simulink model "Template_v3_08_2020a"  (R2020a)
settings: Solver=FixedStepAuto  StartTime=0.0  StopTime=tsim  FixedStep=baseRate  MaxStep=0.0001  RelTol=1e-6  AbsTol=1e-6  EnableMultiTasking=on
values from neighbouring files (symbols this model uses):
  baseRate = 0.05    [Run_Initializer.m]
  drop_states_ARM = [ pi/2, pi/2, 0]    [Run_Initializer.m]
  drop_states_BLACK = [ xLength/2, yLength/2, 0]    [Run_Initializer.m]
  drop_states_BLUE = [ xLength/2-0.5; yLength/2; 0]    [Run_Initializer.m]
  drop_states_RED = [ xLength/2+0.5, yLength/2, pi]    [Run_Initializer.m]
  F_Black_X_nominal = 0.2196    [Run_Initializer.m]
  F_Black_Y_nominal = 0.2825    [Run_Initializer.m]
  F_Blue_X_nominal = 0.2196    [Run_Initializer.m]
  F_Blue_Y_nominal = 0.2825    [Run_Initializer.m]
  F_red_X_nominal = 0.2196    [Run_Initializer.m]
  F_red_Y_nominal = 0.2825    [Run_Initializer.m]
  F_thrusters_BLACK = [F_Black_X_nominal; F_Black_X_nominal;                             F_Black_Y_nominal; F_Black_Y_nominal; F_Black_X_nominal;                              F_Black_X_nominal; F_Black_Y_nominal; F_Black_Y_nominal]    [Run_Initializer.m]
  F_thrusters_BLUE = [F_Blue_X_nominal; F_Blue_X_nominal;                             F_Blue_Y_nominal; F_Blue_Y_nominal; F_Blue_X_nominal;                              F_Blue_X_nominal; F_Blue_Y_nominal; F_Blue_Y_nominal]    [Run_Initializer.m]
  F_thrusters_RED = [F_red_X_nominal; F_red_X_nominal;                             F_red_Y_nominal; F_red_Y_nominal; F_red_X_nominal;                              F_red_X_nominal; F_red_Y_nominal; F_red_Y_nominal]    [Run_Initializer.m]
  Gamma1_el = 0.12    [Run_Initializer.m]
  Gamma1_sh = 0.005    [Run_Initializer.m]
  Gamma1_wr = 0.025    [Run_Initializer.m]
  Gamma2_el = 5    [Run_Initializer.m]
  Gamma2_sh = 15    [Run_Initializer.m]
  Gamma2_wr = 5    [Run_Initializer.m]
  Gamma3_el = 10    [Run_Initializer.m]
  Gamma3_sh = 40    [Run_Initializer.m]
  Gamma3_wr = 40    [Run_Initializer.m]
  Gamma4_el = 0.039    [Run_Initializer.m]
  Gamma4_sh = 0.015    [Run_Initializer.m]
  Gamma4_wr = 0.029    [Run_Initializer.m]
  Gamma5_el = 800    [Run_Initializer.m]
  Gamma5_sh = 800    [Run_Initializer.m]
  Gamma5_wr = 800    [Run_Initializer.m]
  Gamma6_el = 0.000001    (= 1e-06)    [Run_Initializer.m]
  Gamma6_sh = 0.005    [Run_Initializer.m]
  Gamma6_wr = 0.02    [Run_Initializer.m]
  home_states_BLACK = [ xLength/2; yLength/2; 0]    [Run_Initializer.m]
  home_states_BLUE = [ xLength/2-0.9; yLength/2; 0]    [Run_Initializer.m]
  home_states_RED = [ xLength/2+0.9; yLength/2; pi]    [Run_Initializer.m]
  init_states_BLACK = [ xLength/2; yLength/2; 0]    [Run_Initializer.m]
  init_states_BLUE = [ xLength/2-0.9; yLength/2; 0]    [Run_Initializer.m]
  init_states_RED = [ xLength/2+0.9; yLength/2; pi]    [Run_Initializer.m]
  Kd_tb = 1.0    (= 1)    [Run_Initializer.m]
  Kd_tblue = 1    [Run_Initializer.m]
  Kd_tr = 1.0    (= 1)    [Run_Initializer.m]
  Kd_xb = 8    [Run_Initializer.m]
  Kd_xblue = 8    [Run_Initializer.m]
  Kd_xr = 8    [Run_Initializer.m]
  Kd_yb = 8    [Run_Initializer.m]
  Kd_yblue = 8    [Run_Initializer.m]
  Kd_yr = 8    [Run_Initializer.m]
  Kp_tb = 0.1    [Run_Initializer.m]
  Kp_tblue = 0.1    [Run_Initializer.m]
  Kp_tr = 0.1    [Run_Initializer.m]
  Kp_xb = 2    [Run_Initializer.m]
  Kp_xblue = 2    [Run_Initializer.m]
  Kp_xr = 2    [Run_Initializer.m]
  Kp_yb = 2    [Run_Initializer.m]
  Kp_yblue = 2    [Run_Initializer.m]
  Kp_yr = 2    [Run_Initializer.m]
  noise_variance_BLACK = 0    [Run_Initializer.m]
  noise_variance_BLUE = 0    [Run_Initializer.m]
  noise_variance_RED = 0    [Run_Initializer.m]
  Phase0_End = Phase0_Duration    (= 10)    [Run_Initializer.m]
  Phase1_End = Phase0_Duration + Phase1_Duration    (= 15)    [Run_Initializer.m]
  Phase2_End = Phase0_Duration + Phase1_Duration +                                   Phase2_Duration    (= 35)    [Run_Initializer.m]
  Phase3_End = Phase0_Duration + Phase1_Duration +                                   Phase2_Duration + Phase3_Duration    (= 155)    [Run_Initializer.m]
  Phase3_SubPhase1_End = Phase2_End + Phase3_SubPhase1_Duration    (= 155)    [Run_Initializer.m]
  Phase3_SubPhase2_End = Phase2_End + Phase3_SubPhase1_Duration +                                   Phase3_SubPhase2_Duration    (= 155)    [Run_Initializer.m]
  Phase3_SubPhase3_End = Phase2_End + Phase3_SubPhase1_Duration +                                   Phase3_SubPhase2_Duration +                                  Phase3_SubPhase3_Duration    (= 155)    [Run_Initializer.m]
  Phase3_SubPhase4_End = Phase2_End + Phase3_SubPhase1_Duration +                                   Phase3_SubPhase2_Duration +                                  Phase3_SubPhase3_Duration +                                  Phase3_SubPhase4_Duration    [Run_Initializer.m]
  Phase4_End = Phase0_Duration + Phase1_Duration +                                   Phase2_Duration + Phase3_Duration +                                   Phase4_Duration    (= 275)    [Run_Initializer.m]
  Phase5_End = Phase0_Duration + Phase1_Duration +                                   Phase2_Duration + Phase3_Duration +                                   Phase4_Duration + Phase5_Duration    (= 295)    [Run_Initializer.m]
  thruster_dist2CG_BLACK = [72.80;-65.20;61.75;-79.75;65.20;-65.20;74.25;-54.75]    [Run_Initializer.m]
  thruster_dist2CG_BLUE = [83.10;-54.90;71.50;-70.00;54.90;-75.50;64.50;-64.50]    [Run_Initializer.m]
  thruster_dist2CG_RED = [69.38;-56.62;50.01;-81.49;61.12;-68.38;78.99;-52.01]    [Run_Initializer.m]
  Tz_lim_elarm = .1    (= 0.1)    [Run_Initializer.m]
  Tz_lim_sharm = .1    (= 0.1)    [Run_Initializer.m]
  Tz_lim_wrarm = .1    (= 0.1)    [Run_Initializer.m]
  xLength = 3.51155    [Run_Initializer.m]
  yLength = 2.41935    [Run_Initializer.m]
undefined symbols (not defined in the file or in its folder): b0, b1, b_out, CHASER_ABSOLUTE_POSITION, DiscIntNeverNeededParam, MAX_BODY_ANGULAR_VELOCITY, MAX_VELOCITY, model_param, platformSelection, relevant_half_range, relevant_state_mean, serverRate, simMode, w0, w1, w_out
libraries: dspstat3 x18, raspberrypiBasiclib x9, dspsigops x9, embdlinuxlib x7, simulink x7, MainLibrary x4, mspfiltlib x3, dsparch4 x3, etargetslib x1, sensehatlib x1
(part 5 of 12)

== system Template_v3_08_2020a/Phase #2: Move to Initial Position/Change RED Behavior/RED+ARM ==
  note: ARM Control Law - RED
  note: This section is reserved for any control law for the robotic manipulator.
  Action Port : ActionPort  ActionPortLabel=if(u1 == 4 | u1 == 5 | u1 == 10 | u1 == 11)
  Constant4 : Constant  Value=pi/2
  Constant5 : Constant  Value=pi/2
  Constant6 : Constant  Value=0
  Constant7 : Constant
  Data Store Write : DataStoreWrite  DataStoreName=RED_Shoulder_Command
  Data Store Write1 : DataStoreWrite  DataStoreName=RED_Elbow_Command
  Data Store Write2 : DataStoreWrite  DataStoreName=RED_Wrist_Command
  Data Store Write3 : DataStoreWrite  DataStoreName=RED_ARM_Control_Mode
  wires:
  Constant7/1 -> Data Store Write3/1
  Constant5/1 -> Data Store Write1/1
  Constant4/1 -> Data Store Write/1
  Constant6/1 -> Data Store Write2/1

== system Template_v3_08_2020a/Phase #3: Experiment/Change BLACK Behavior/Sub-Phase #1 ==
  note: PD Control Law - BLACK
  note: Additional Blocks
  note: A simple PD control law is used here to command the platform to it's initial position, as defined in the initializer.
  note: Additional blocks are stored here.
  Action Port : ActionPort  ActionPortLabel=if(u1 < u2)
  BLACK_Fx : DataStoreWrite  DataStoreName=BLACK_Fx
  BLACK_Fy : DataStoreWrite  DataStoreName=BLACK_Fy
  BLACK_Px : DataStoreRead  DataStoreName=BLACK_Px
  "BLACK_Py " : DataStoreRead  DataStoreName=BLACK_Py
  BLACK_Rz : DataStoreRead  DataStoreName=BLACK_Rz
  BLACK_RzD1 : Subsystem
  BLACK_Tz : DataStoreWrite  DataStoreName=BLACK_Tz
  Custom Discrete PD (Attitude) : Subsystem
  Custom Discrete PD (X-Position) : Subsystem
  Custom Discrete PD (Y-Position) : Subsystem
  Data Store Write3 : DataStoreWrite  DataStoreName=Float_State
  Desired X-Position (BLACK) : Constant  Value=xLength/2  SampleTime=-1
  Desired Y-Position (BLACK) : Constant  Value=yLength/2  SampleTime=-1
  Hough Control : Subsystem
  Puck State : Constant
  Subtract : Sum  Inputs=+-
  Subtract1 : Sum  Inputs=+-
  wires:
  Puck State/1 -> Data Store Write3/1
  "BLACK_Py "/1 -> Subtract1/2
  Desired X-Position (BLACK)/1 -> Subtract/1
  BLACK_RzD1/1(Out1) -> Hough Control/1(Ref)
  Custom Discrete PD (X-Position)/1(Fx) -> BLACK_Fx/1
  Desired Y-Position (BLACK)/1 -> Subtract1/1
  Hough Control/1(Err) -> Custom Discrete PD (Attitude)/1(ez)
  Subtract/1 -> Custom Discrete PD (X-Position)/1(ex)
  Custom Discrete PD (Y-Position)/1(Fy) -> BLACK_Fy/1
  Subtract1/1 -> Custom Discrete PD (Y-Position)/1(ey)
  Custom Discrete PD (Attitude)/1(Tz) -> BLACK_Tz/1
  BLACK_Rz/1 -> Hough Control/2(Act)
  BLACK_Px/1 -> Subtract/2

== system Template_v3_08_2020a/Phase #3: Experiment/Change BLACK Behavior/Sub-Phase #2  ==
  note: PD Control Law - BLACK
  note: Additional Blocks
  note: Additional blocks are stored here.
  Action Port : ActionPort  ActionPortLabel=elseif(u1 < u3)
  BLACK_Fx : DataStoreWrite  DataStoreName=BLACK_Fx
  BLACK_Fy : DataStoreWrite  DataStoreName=BLACK_Fy
  BLACK_Px : DataStoreRead  DataStoreName=BLACK_Px
  "BLACK_Py " : DataStoreRead  DataStoreName=BLACK_Py
  BLACK_Rz : DataStoreRead  DataStoreName=BLACK_Rz
  BLACK_RzD1 : Subsystem
  BLACK_Tz : DataStoreWrite  DataStoreName=BLACK_Tz
  Custom Discrete PD (Attitude) : Subsystem
  Custom Discrete PD (X-Position) : Subsystem
  Custom Discrete PD (Y-Position) : Subsystem
  Data Store Write3 : DataStoreWrite  DataStoreName=Float_State
  Desired X-Position (BLACK) : Constant  Value=xLength/2  SampleTime=-1
  Desired Y-Position (BLACK) : Constant  Value=yLength/2  SampleTime=-1
  Hough Control : Subsystem
  Puck State : Constant
  Subtract : Sum  Inputs=+-
  Subtract1 : Sum  Inputs=+-
  wires:
  Puck State/1 -> Data Store Write3/1
  BLACK_Px/1 -> Subtract/2
  Custom Discrete PD (Y-Position)/1(Fy) -> BLACK_Fy/1
  Subtract/1 -> Custom Discrete PD (X-Position)/1(ex)
  Desired Y-Position (BLACK)/1 -> Subtract1/1
  Custom Discrete PD (Attitude)/1(Tz) -> BLACK_Tz/1
  Subtract1/1 -> Custom Discrete PD (Y-Position)/1(ey)
  BLACK_Rz/1 -> Hough Control/2(Act)
  Custom Discrete PD (X-Position)/1(Fx) -> BLACK_Fx/1
  Hough Control/1(Err) -> Custom Discrete PD (Attitude)/1(ez)
  "BLACK_Py "/1 -> Subtract1/2
  Desired X-Position (BLACK)/1 -> Subtract/1
  BLACK_RzD1/1(Out1) -> Hough Control/1(Ref)

== system Template_v3_08_2020a/Phase #3: Experiment/Change BLACK Behavior/Sub-Phase #3  ==
  note: PD Control Law - BLACK
  note: Additional Blocks
  note: Additional blocks are stored here.
  Action Port : ActionPort  ActionPortLabel=elseif( u1 < u4)
  BLACK_Fx : DataStoreWrite  DataStoreName=BLACK_Fx
  BLACK_Fy : DataStoreWrite  DataStoreName=BLACK_Fy
  BLACK_Px : DataStoreRead  DataStoreName=BLACK_Px
  "BLACK_Py " : DataStoreRead  DataStoreName=BLACK_Py
  BLACK_Rz : DataStoreRead  DataStoreName=BLACK_Rz
  BLACK_RzD1 : Subsystem
  BLACK_Tz : DataStoreWrite  DataStoreName=BLACK_Tz
  Custom Discrete PD (Attitude) : Subsystem
  Custom Discrete PD (X-Position) : Subsystem
  Custom Discrete PD (Y-Position) : Subsystem
  Data Store Write3 : DataStoreWrite  DataStoreName=Float_State
  Desired X-Position (BLACK) : Constant  Value=xLength/2  SampleTime=-1
  Desired Y-Position (BLACK) : Constant  Value=yLength/2  SampleTime=-1
  Hough Control : Subsystem
  Puck State : Constant
  Subtract : Sum  Inputs=+-
  Subtract1 : Sum  Inputs=+-
  wires:
  Puck State/1 -> Data Store Write3/1
  BLACK_Px/1 -> Subtract/2
  Custom Discrete PD (Y-Position)/1(Fy) -> BLACK_Fy/1
  Subtract/1 -> Custom Discrete PD (X-Position)/1(ex)
  Desired Y-Position (BLACK)/1 -> Subtract1/1
  Custom Discrete PD (Attitude)/1(Tz) -> BLACK_Tz/1
  Subtract1/1 -> Custom Discrete PD (Y-Position)/1(ey)
  BLACK_Rz/1 -> Hough Control/2(Act)
  Custom Discrete PD (X-Position)/1(Fx) -> BLACK_Fx/1
  Hough Control/1(Err) -> Custom Discrete PD (Attitude)/1(ez)
  "BLACK_Py "/1 -> Subtract1/2
  Desired X-Position (BLACK)/1 -> Subtract/1
  BLACK_RzD1/1(Out1) -> Hough Control/1(Ref)

== system Template_v3_08_2020a/Phase #3: Experiment/Change BLACK Behavior/Sub-Phase #4 ==
  note: PD Control Law - BLACK
  note: Additional Blocks
  note: A simple PD control law is used here to command the platform to it's initial position, as defined in the initializer.
  note: Additional blocks are stored here.
  Action Port : ActionPort  ActionPortLabel=elseif( u1 < u5)
  BLACK_Fx : DataStoreWrite  DataStoreName=BLACK_Fx
  BLACK_Fy : DataStoreWrite  DataStoreName=BLACK_Fy
  BLACK_Px : DataStoreRead  DataStoreName=BLACK_Px
  "BLACK_Py " : DataStoreRead  DataStoreName=BLACK_Py
  BLACK_Rz : DataStoreRead  DataStoreName=BLACK_Rz
  BLACK_RzD : Subsystem  Commented=on
  BLACK_RzD1 : Subsystem
  BLACK_Tz : DataStoreWrite  DataStoreName=BLACK_Tz
  Custom Discrete PD (Attitude) : Subsystem
  Custom Discrete PD (X-Position) : Subsystem
  Custom Discrete PD (Y-Position) : Subsystem
  Data Store Write3 : DataStoreWrite  DataStoreName=Float_State
  Desired X-Position (BLACK) : Constant  Value=xLength/2  SampleTime=-1
  Desired Y-Position (BLACK) : Constant  Value=yLength/2  SampleTime=-1
  Hough Control : Subsystem
  Puck State : Constant
  Subtract : Sum  Inputs=+-
  Subtract1 : Sum  Inputs=+-
  wires:
  Puck State/1 -> Data Store Write3/1
  BLACK_Px/1 -> Subtract/2
  Custom Discrete PD (Y-Position)/1(Fy) -> BLACK_Fy/1
  Subtract/1 -> Custom Discrete PD (X-Position)/1(ex)
  Desired Y-Position (BLACK)/1 -> Subtract1/1
  Custom Discrete PD (Attitude)/1(Tz) -> BLACK_Tz/1
  Subtract1/1 -> Custom Discrete PD (Y-Position)/1(ey)
  BLACK_Rz/1 -> Hough Control/2(Act)
  Custom Discrete PD (X-Position)/1(Fx) -> BLACK_Fx/1
  Hough Control/1(Err) -> Custom Discrete PD (Attitude)/1(ez)
  "BLACK_Py "/1 -> Subtract1/2
  Desired X-Position (BLACK)/1 -> Subtract/1
  BLACK_RzD1/1(Out1) -> Hough Control/1(Ref)

== system Template_v3_08_2020a/Phase #3: Experiment/Change BLACK Behavior/Subsystem ==
  Universal_Time : DataStoreRead  DataStoreName=Univ_Time
  Time : Outport  VectorParamsAs1DForOutWhenUnconnected=off
  wires:
  Universal_Time/1 -> Time/1

== system Template_v3_08_2020a/Phase #3: Experiment/Change BLUE Behavior/Sub-Phase #1 ==
  note: PD Control Law - BLUE
  note: A simple PD control law is used here to command the platform to it's initial position, as defined in the initializer.
  note: Additional Blocks
  note: Additional blocks are stored here.
  Action Port : ActionPort  ActionPortLabel=if(u1 < u2)
  BLUE_Fx : DataStoreWrite  DataStoreName=BLUE_Fx
  BLUE_Fy : DataStoreWrite  DataStoreName=BLUE_Fy
  BLUE_Px : DataStoreRead  DataStoreName=BLUE_Px
  "BLUE_Py " : DataStoreRead  DataStoreName=BLUE_Py
  BLUE_Rz : DataStoreRead  DataStoreName=BLUE_Rz
  BLUE_Tz : DataStoreWrite  DataStoreName=BLUE_Tz
  Custom Discrete PD (Attitude) : Subsystem
  Custom Discrete PD (X-Position) : Subsystem
  Custom Discrete PD (Y-Position) : Subsystem
  Data Store Write1 : DataStoreWrite  DataStoreName=Float_State
  Hough Control : Subsystem
  MATLAB Function2 : MATLAB Function  TreatAsAtomicUnit=on
  MATLAB Function3 : MATLAB Function  TreatAsAtomicUnit=on
  Puck State : Constant
  RED_Rz_REF1 : Subsystem
  Subsystem2 : Subsystem
  Subtract : Sum  Inputs=+-
  Subtract1 : Sum  Inputs=+-
  wires:
  Puck State/1 -> Data Store Write1/1
  Subtract/1 -> Custom Discrete PD (X-Position)/1(ex)
  Custom Discrete PD (X-Position)/1(Fx) -> BLUE_Fx/1
  Subtract1/1 -> Custom Discrete PD (Y-Position)/1(ey)
  Hough Control/1(Err) -> Custom Discrete PD (Attitude)/1(ez)
  Custom Discrete PD (Attitude)/1(Tz) -> BLUE_Tz/1
  Custom Discrete PD (Y-Position)/1(Fy) -> BLUE_Fy/1
  MATLAB Function3/1(y) -> Subtract1/1
  BLUE_Px/1 -> Subtract/2
  MATLAB Function2/1(x) -> Subtract/1
  Subsystem2/1(Out1) -> MATLAB Function2/1(t), MATLAB Function3/1(t)
  "BLUE_Py "/1 -> Subtract1/2
  RED_Rz_REF1/1(Ref) -> Hough Control/1(Ref)
  BLUE_Rz/1 -> Hough Control/2(Act)

== system Template_v3_08_2020a/Phase #3: Experiment/Change BLUE Behavior/Sub-Phase #2  ==
  note: Additional blocks are stored here.
  note: A simple PD control law is used here to command the platform to it's initial position, as defined in the initializer.
  note: Additional Blocks
  note: PD Control Law - BLUE
  Action Port : ActionPort  ActionPortLabel=elseif(u1 < u3)
  BLUE_Fx : DataStoreWrite  DataStoreName=BLUE_Fx
  BLUE_Fy : DataStoreWrite  DataStoreName=BLUE_Fy
  BLUE_Px : DataStoreRead  DataStoreName=BLUE_Px
  "BLUE_Py " : DataStoreRead  DataStoreName=BLUE_Py
  BLUE_Rz : DataStoreRead  DataStoreName=BLUE_Rz
  BLUE_Tz : DataStoreWrite  DataStoreName=BLUE_Tz
  Custom Discrete PD (Attitude) : Subsystem
  Custom Discrete PD (X-Position) : Subsystem
  Custom Discrete PD (Y-Position) : Subsystem
  Data Store Write1 : DataStoreWrite  DataStoreName=Float_State
  Hough Control : Subsystem
  MATLAB Function2 : MATLAB Function  TreatAsAtomicUnit=on
  MATLAB Function3 : MATLAB Function  TreatAsAtomicUnit=on
  Puck State : Constant
  RED_Rz_REF1 : Subsystem
  Subsystem2 : Subsystem
  Subtract : Sum  Inputs=+-
  Subtract1 : Sum  Inputs=+-
  wires:
  Puck State/1 -> Data Store Write1/1
  BLUE_Rz/1 -> Hough Control/2(Act)
  RED_Rz_REF1/1(Ref) -> Hough Control/1(Ref)
  Custom Discrete PD (Y-Position)/1(Fy) -> BLUE_Fy/1
  Subtract/1 -> Custom Discrete PD (X-Position)/1(ex)
  Subtract1/1 -> Custom Discrete PD (Y-Position)/1(ey)
  BLUE_Px/1 -> Subtract/2
  Custom Discrete PD (X-Position)/1(Fx) -> BLUE_Fx/1
  "BLUE_Py "/1 -> Subtract1/2
  Subsystem2/1(Out1) -> MATLAB Function2/1(t), MATLAB Function3/1(t)
  MATLAB Function2/1(x) -> Subtract/1
  Hough Control/1(Err) -> Custom Discrete PD (Attitude)/1(ez)
  MATLAB Function3/1(y) -> Subtract1/1
  Custom Discrete PD (Attitude)/1(Tz) -> BLUE_Tz/1

== system Template_v3_08_2020a/Phase #3: Experiment/Change BLUE Behavior/Sub-Phase #3  ==
  note: Additional blocks are stored here.
  note: A simple PD control law is used here to command the platform to it's initial position, as defined in the initializer.
  note: Additional Blocks
  note: PD Control Law - BLUE
  Action Port : ActionPort  ActionPortLabel=elseif( u1 < u4)
  BLUE_Fx : DataStoreWrite  DataStoreName=BLUE_Fx
  BLUE_Fy : DataStoreWrite  DataStoreName=BLUE_Fy
  BLUE_Px : DataStoreRead  DataStoreName=BLUE_Px
  "BLUE_Py " : DataStoreRead  DataStoreName=BLUE_Py
  BLUE_Rz : DataStoreRead  DataStoreName=BLUE_Rz
  BLUE_Tz : DataStoreWrite  DataStoreName=BLUE_Tz
  Custom Discrete PD (Attitude) : Subsystem
  Custom Discrete PD (X-Position) : Subsystem
  Custom Discrete PD (Y-Position) : Subsystem
  Data Store Write1 : DataStoreWrite  DataStoreName=Float_State
  Hough Control : Subsystem
  MATLAB Function2 : MATLAB Function  TreatAsAtomicUnit=on
  MATLAB Function3 : MATLAB Function  TreatAsAtomicUnit=on
  Puck State : Constant
  RED_Rz_REF1 : Subsystem
  Subsystem2 : Subsystem
  Subtract : Sum  Inputs=+-
  Subtract1 : Sum  Inputs=+-
  wires:
  Puck State/1 -> Data Store Write1/1
  BLUE_Rz/1 -> Hough Control/2(Act)
  RED_Rz_REF1/1(Ref) -> Hough Control/1(Ref)
  Custom Discrete PD (Y-Position)/1(Fy) -> BLUE_Fy/1
  Subtract/1 -> Custom Discrete PD (X-Position)/1(ex)
  Subtract1/1 -> Custom Discrete PD (Y-Position)/1(ey)
  BLUE_Px/1 -> Subtract/2
  Custom Discrete PD (X-Position)/1(Fx) -> BLUE_Fx/1
  "BLUE_Py "/1 -> Subtract1/2
  Subsystem2/1(Out1) -> MATLAB Function2/1(t), MATLAB Function3/1(t)
  MATLAB Function2/1(x) -> Subtract/1
  Hough Control/1(Err) -> Custom Discrete PD (Attitude)/1(ez)
  MATLAB Function3/1(y) -> Subtract1/1
  Custom Discrete PD (Attitude)/1(Tz) -> BLUE_Tz/1

== system Template_v3_08_2020a/Phase #3: Experiment/Change BLUE Behavior/Sub-Phase #4 ==
  note: Additional blocks are stored here.
  note: A simple PD control law is used here to command the platform to it's initial position, as defined in the initializer.
  note: Additional Blocks
  note: PD Control Law - BLUE
  Action Port : ActionPort  ActionPortLabel=elseif( u1 < u5)
  BLUE_Fx : DataStoreWrite  DataStoreName=BLUE_Fx
  BLUE_Fy : DataStoreWrite  DataStoreName=BLUE_Fy
  BLUE_Px : DataStoreRead  DataStoreName=BLUE_Px
  "BLUE_Py " : DataStoreRead  DataStoreName=BLUE_Py
  BLUE_Rz : DataStoreRead  DataStoreName=BLUE_Rz
  BLUE_Tz : DataStoreWrite  DataStoreName=BLUE_Tz
  Custom Discrete PD (Attitude) : Subsystem
  Custom Discrete PD (X-Position) : Subsystem
  Custom Discrete PD (Y-Position) : Subsystem
  Data Store Write1 : DataStoreWrite  DataStoreName=Float_State
  Hough Control : Subsystem
  MATLAB Function2 : MATLAB Function  TreatAsAtomicUnit=on
  MATLAB Function3 : MATLAB Function  TreatAsAtomicUnit=on
  Puck State : Constant
  RED_Rz_REF1 : Subsystem
  Subsystem2 : Subsystem
  Subtract : Sum  Inputs=+-
  Subtract1 : Sum  Inputs=+-
  wires:
  Puck State/1 -> Data Store Write1/1
  BLUE_Rz/1 -> Hough Control/2(Act)
  RED_Rz_REF1/1(Ref) -> Hough Control/1(Ref)
  Custom Discrete PD (Y-Position)/1(Fy) -> BLUE_Fy/1
  Subtract/1 -> Custom Discrete PD (X-Position)/1(ex)
  Subtract1/1 -> Custom Discrete PD (Y-Position)/1(ey)
  BLUE_Px/1 -> Subtract/2
  Custom Discrete PD (X-Position)/1(Fx) -> BLUE_Fx/1
  "BLUE_Py "/1 -> Subtract1/2
  Subsystem2/1(Out1) -> MATLAB Function2/1(t), MATLAB Function3/1(t)
  MATLAB Function2/1(x) -> Subtract/1
  Hough Control/1(Err) -> Custom Discrete PD (Attitude)/1(ez)
  MATLAB Function3/1(y) -> Subtract1/1
  Custom Discrete PD (Attitude)/1(Tz) -> BLUE_Tz/1

== system Template_v3_08_2020a/Phase #3: Experiment/Change BLUE Behavior/Subsystem ==
  Universal_Time : DataStoreRead  DataStoreName=Univ_Time
  Time : Outport  VectorParamsAs1DForOutWhenUnconnected=off
  wires:
  Universal_Time/1 -> Time/1

== system Template_v3_08_2020a/Phase #3: Experiment/Change RED Behavior/Sub-Phase #1 ==
  note: PD Control Law - RED
  note: Additional Blocks
  note: Additional blocks are stored above. Note that to control attitude using the RW, simply replace RED_Tz with RED_Tz_RW.
  note: A simple PD control law is used here to command the platform to it's initial position, as defined in the initializer.
  note: ARM Control Law - RED
  Action Port : ActionPort  ActionPortLabel=if(u1 < u2)
  Constant1 : Constant  Value=0
  Constant4 : Constant  Value=platformSelection
  Custom Discrete PD (Attitude) : Subsystem
  Custom Discrete PD (X-Position) : Subsystem
  Custom Discrete PD (Y-Position) : Subsystem
  Data Store Write3 : DataStoreWrite  DataStoreName=Float_State
  Hough Control : Subsystem
  If : If  IfExpression=u1 == 4 | u1 == 5 | u1 == 10 | u1 == 11
  MATLAB Function : MATLAB Function  TreatAsAtomicUnit=on
  MATLAB Function1 : MATLAB Function  TreatAsAtomicUnit=on
  Puck State : Constant
  RED : Subsystem  TreatAsAtomicUnit=on
  RED+ARM : Subsystem  TreatAsAtomicUnit=on
  RED_Fx : DataStoreWrite  DataStoreName=RED_Fx
  RED_Fy : DataStoreWrite  DataStoreName=RED_Fy
  RED_Px3 : DataStoreRead  DataStoreName=RED_Px
  "RED_Py " : DataStoreRead  DataStoreName=RED_Py
  RED_Rz : DataStoreRead  DataStoreName=RED_Rz
  RED_RzD : Subsystem
  RED_Tz : DataStoreWrite  DataStoreName=RED_Tz
  RED_Tz_RW : DataStoreWrite  DataStoreName=RED_Tz_RW
  Subsystem1 : Subsystem
  Subtract : Sum  Inputs=+-
  Subtract1 : Sum  Inputs=+-
  wires:
  Constant1/1 -> RED_Tz_RW/1
  Puck State/1 -> Data Store Write3/1
  Custom Discrete PD (Y-Position)/1(Fy) -> RED_Fy/1
  Custom Discrete PD (X-Position)/1(Fx) -> RED_Fx/1
  Custom Discrete PD (Attitude)/1(Tz) -> RED_Tz/1
  Hough Control/1(Err) -> Custom Discrete PD (Attitude)/1(ez)
  Subsystem1/1(Out1) -> MATLAB Function/1(t), MATLAB Function1/1(t)
  RED_Px3/1 -> Subtract/2
  MATLAB Function1/1(y) -> Subtract1/1
  "RED_Py "/1 -> Subtract1/2
  MATLAB Function/1(x) -> Subtract/1
  Subtract/1 -> Custom Discrete PD (X-Position)/1(ex)
  RED_Rz/1 -> Hough Control/2(Act)
  Subtract1/1 -> Custom Discrete PD (Y-Position)/1(ey)
  RED_RzD/1(Ref) -> Hough Control/1(Ref)
  If/1 -> RED+ARM/Action
  Constant4/1 -> If/1
  If/2 -> RED/Action

== system Template_v3_08_2020a/Phase #3: Experiment/Change RED Behavior/Sub-Phase #2  ==
  note: PD Control Law - RED
  note: Additional Blocks
  note: Additional blocks are stored above. Note that to control attitude using the RW, simply replace RED_Tz with RED_Tz_RW.
  note: ARM Control Law - RED
  Action Port : ActionPort  ActionPortLabel=elseif(u1 < u3)
  BLACK_RzD1 : Subsystem
  Constant1 : Constant  Value=0
  Constant4 : Constant  Value=platformSelection
  Custom Discrete PD (Attitude) : Subsystem
  Custom Discrete PD (X-Position) : Subsystem
  Custom Discrete PD (Y-Position) : Subsystem
  Data Store Write3 : DataStoreWrite  DataStoreName=Float_State
  Hough Control : Subsystem
  If : If  IfExpression=u1 == 4 | u1 == 5 | u1 == 10 | u1 == 11
  MATLAB Function : MATLAB Function  TreatAsAtomicUnit=on
  MATLAB Function1 : MATLAB Function  TreatAsAtomicUnit=on
  Puck State : Constant
  RED : Subsystem  TreatAsAtomicUnit=on
  RED+ARM : Subsystem  TreatAsAtomicUnit=on
  RED_Fx : DataStoreWrite  DataStoreName=RED_Fx
  RED_Fy : DataStoreWrite  DataStoreName=RED_Fy
  RED_Px1 : DataStoreRead  DataStoreName=RED_Px
  "RED_Py " : DataStoreRead  DataStoreName=RED_Py
  RED_Rz : DataStoreRead  DataStoreName=RED_Rz
  RED_Tz : DataStoreWrite  DataStoreName=RED_Tz
  RED_Tz_RW : DataStoreWrite  DataStoreName=RED_Tz_RW
  Subsystem1 : Subsystem
  Subtract : Sum  Inputs=+-
  Subtract2 : Sum  Inputs=+-
  wires:
  Constant1/1 -> RED_Tz_RW/1
  Puck State/1 -> Data Store Write3/1
  Subtract2/1 -> Custom Discrete PD (Y-Position)/1(ey)
  "RED_Py "/1 -> Subtract2/2
  BLACK_RzD1/1(Ref) -> Hough Control/1(Ref)
  MATLAB Function/1(x) -> Subtract/1
  RED_Rz/1 -> Hough Control/2(Act)
  Subtract/1 -> Custom Discrete PD (X-Position)/1(ex)
  MATLAB Function1/1(y) -> Subtract2/1
  Custom Discrete PD (Attitude)/1(Tz) -> RED_Tz/1
  RED_Px1/1 -> Subtract/2
  Subsystem1/1(Out1) -> MATLAB Function/1(t), MATLAB Function1/1(t)
  Custom Discrete PD (X-Position)/1(Fx) -> RED_Fx/1
  Hough Control/1(Err) -> Custom Discrete PD (Attitude)/1(ez)
  Custom Discrete PD (Y-Position)/1(Fy) -> RED_Fy/1
  If/1 -> RED+ARM/Action
  Constant4/1 -> If/1
  If/2 -> RED/Action

== system Template_v3_08_2020a/Phase #3: Experiment/Change RED Behavior/Sub-Phase #3  ==
  note: PD Control Law - RED
  note: Additional Blocks
  note: Additional blocks are stored above. Note that to control attitude using the RW, simply replace RED_Tz with RED_Tz_RW.
  note: ARM Control Law - RED
  Action Port : ActionPort  ActionPortLabel=elseif( u1 < u4)
  Constant1 : Constant  Value=platformSelection
  Constant4 : Constant  Value=0
  Custom Discrete PD (Attitude) : Subsystem  Commented=on
  Custom Discrete PD (X-Position) : Subsystem
  Custom Discrete PD (Y-Position) : Subsystem
  Data Store Write3 : DataStoreWrite  DataStoreName=Float_State
  Hough Control : Subsystem  Commented=on
  If : If  IfExpression=u1 == 4 | u1 == 5 | u1 == 10 | u1 == 11
  MATLAB Function : MATLAB Function  TreatAsAtomicUnit=on
  MATLAB Function1 : MATLAB Function  TreatAsAtomicUnit=on
  Puck State : Constant
  RED : Subsystem  TreatAsAtomicUnit=on
  RED+ARM : Subsystem  TreatAsAtomicUnit=on
  RED_Fx : DataStoreWrite  DataStoreName=RED_Fx
  RED_Fy : DataStoreWrite  DataStoreName=RED_Fy
  RED_Px1 : DataStoreRead  DataStoreName=RED_Px
  "RED_Py " : DataStoreRead  DataStoreName=RED_Py
  RED_Rz : DataStoreRead  Commented=on  DataStoreName=RED_Rz
  RED_Rz_REF : Subsystem  Commented=on
  RED_Tz : DataStoreWrite  Commented=on  DataStoreName=RED_Tz
  RED_Tz_RW : DataStoreWrite  DataStoreName=RED_Tz_RW
  Saturation : Saturate  UpperLimit=Tz_lim_sharm  LowerLimit=-Tz_lim_sharm
  Saturation1 : Saturate  UpperLimit=Tz_lim_elarm  LowerLimit=-Tz_lim_elarm
  Saturation3 : Saturate  UpperLimit=Tz_lim_wrarm  LowerLimit=-Tz_lim_wrarm
  Subsystem1 : Subsystem
  Subtract : Sum  Inputs=+-
  Subtract2 : Sum  Inputs=+-
  wires:
  Puck State/1 -> Data Store Write3/1
  Hough Control/1(Err) -> Custom Discrete PD (Attitude)/1(ez)
  Custom Discrete PD (Y-Position)/1(Fy) -> RED_Fy/1
  Custom Discrete PD (X-Position)/1(Fx) -> RED_Fx/1
  RED_Rz/1 -> Hough Control/2(Act)
  MATLAB Function1/1(y) -> Subtract2/1
  Custom Discrete PD (Attitude)/1(Tz) -> RED_Tz/1
  MATLAB Function/1(x) -> Subtract/1
  Subtract/1 -> Custom Discrete PD (X-Position)/1(ex)
  "RED_Py "/1 -> Subtract2/2
  RED_Rz_REF/1(Ref) -> Hough Control/1(Ref)
  RED_Px1/1 -> Subtract/2
  Subsystem1/1(Out1) -> MATLAB Function/1(t), MATLAB Function1/1(t)
  Subtract2/1 -> Custom Discrete PD (Y-Position)/1(ey)
  Constant4/1 -> RED_Tz_RW/1
  If/1 -> RED+ARM/Action
  Constant1/1 -> If/1
  If/2 -> RED/Action

== system Template_v3_08_2020a/Phase #3: Experiment/Change RED Behavior/Sub-Phase #4 ==
  note: PD Control Law - RED
  note: Additional Blocks
  note: Additional blocks are stored above. Note that to control attitude using the RW, simply replace RED_Tz with RED_Tz_RW.
  note: A simple PD control law is used here to command the platform to it's initial position, as defined in the initializer.
  note: ARM Control Law - RED
  Action Port : ActionPort  ActionPortLabel=elseif( u1 < u5)
  Constant1 : Constant  Value=0
  Constant3 : Constant  Value=platformSelection
  Custom Discrete PD (Attitude) : Subsystem
  Custom Discrete PD (X-Position) : Subsystem
  Custom Discrete PD (Y-Position) : Subsystem
  Data Store Write3 : DataStoreWrite  DataStoreName=Float_State
  Hough Control : Subsystem
  If : If  IfExpression=u1 == 4 | u1 == 5 | u1 == 10 | u1 == 11
  MATLAB Function : MATLAB Function  TreatAsAtomicUnit=on
  MATLAB Function1 : MATLAB Function  TreatAsAtomicUnit=on
  Puck State : Constant
  RED : Subsystem  TreatAsAtomicUnit=on
  RED+ARM : Subsystem  TreatAsAtomicUnit=on
  RED_Fx : DataStoreWrite  DataStoreName=RED_Fx
  RED_Fy : DataStoreWrite  DataStoreName=RED_Fy
  RED_Px1 : DataStoreRead  DataStoreName=RED_Px
  "RED_Py " : DataStoreRead  DataStoreName=RED_Py
  RED_Rz : DataStoreRead  DataStoreName=RED_Rz
  RED_Rz_REF : Subsystem
  RED_Tz : DataStoreWrite  DataStoreName=RED_Tz
  RED_Tz_RW : DataStoreWrite  DataStoreName=RED_Tz_RW
  Subsystem1 : Subsystem
  Subtract : Sum  Inputs=+-
  Subtract1 : Sum  Inputs=+-
  wires:
  Constant1/1 -> RED_Tz_RW/1
  RED_Rz/1 -> Hough Control/2(Act)
  Subtract/1 -> Custom Discrete PD (X-Position)/1(ex)
  Custom Discrete PD (X-Position)/1(Fx) -> RED_Fx/1
  Custom Discrete PD (Y-Position)/1(Fy) -> RED_Fy/1
  RED_Px1/1 -> Subtract/2
  Custom Discrete PD (Attitude)/1(Tz) -> RED_Tz/1
  "RED_Py "/1 -> Subtract1/2
  Hough Control/1(Err) -> Custom Discrete PD (Attitude)/1(ez)
  Subtract1/1 -> Custom Discrete PD (Y-Position)/1(ey)
  Puck State/1 -> Data Store Write3/1
  Subsystem1/1(Out1) -> MATLAB Function/1(t), MATLAB Function1/1(t)
  MATLAB Function/1(x) -> Subtract/1
  MATLAB Function1/1(y) -> Subtract1/1
  RED_Rz_REF/1(Ref) -> Hough Control/1(Ref)
  If/2 -> RED/Action
  If/1 -> RED+ARM/Action
  Constant3/1 -> If/1

== system Template_v3_08_2020a/Phase #3: Experiment/Change RED Behavior/Subsystem ==
  Universal_Time : DataStoreRead  DataStoreName=Univ_Time
  Time : Outport  VectorParamsAs1DForOutWhenUnconnected=off
  wires:
  Universal_Time/1 -> Time/1

== system Template_v3_08_2020a/Phase #4: Return Home/Change BLACK Behavior/Custom Discrete PD (Attitude) ==
  ez : Inport
  Sum3 : Sum
  kd_tb : Gain  Gain=Kd_tb
  kp_tb : Gain  Gain=Kp_tb
  "x_dot -> x1" : Subsystem
  Tz : Outport  VectorParamsAs1DForOutWhenUnconnected=off
  wires:
  kd_tb/1 -> Sum3/1
  Sum3/1 -> Tz/1
  kp_tb/1 -> Sum3/2
  "x_dot -> x1"/1(dy(t)/dt) -> kd_tb/1
  ez/1 -> "x_dot -> x1"/1(y(t)), kp_tb/1

== system Template_v3_08_2020a/Phase #4: Return Home/Change BLACK Behavior/Custom Discrete PD (X-Position) ==
  ex : Inport
  Sum3 : Sum
  kd_xb : Gain  Gain=Kd_xb
  kp_xb : Gain  Gain=Kp_xb
  "x_dot -> x1" : Subsystem
  Fx : Outport  VectorParamsAs1DForOutWhenUnconnected=off
  wires:
  kd_xb/1 -> Sum3/1
  ex/1 -> "x_dot -> x1"/1(y(t)), kp_xb/1
  kp_xb/1 -> Sum3/2
  "x_dot -> x1"/1(dy(t)/dt) -> kd_xb/1
  Sum3/1 -> Fx/1

== system Template_v3_08_2020a/Phase #4: Return Home/Change BLACK Behavior/Custom Discrete PD (Y-Position) ==
  ey : Inport
  Sum3 : Sum
  kd_yb : Gain  Gain=Kd_yb
  kp_yb : Gain  Gain=Kp_yb
  "x_dot -> x1" : Subsystem
  Fy : Outport  VectorParamsAs1DForOutWhenUnconnected=off
  wires:
  kd_yb/1 -> Sum3/1
  Sum3/1 -> Fy/1
  kp_yb/1 -> Sum3/2
  "x_dot -> x1"/1(dy(t)/dt) -> kd_yb/1
  ey/1 -> "x_dot -> x1"/1(y(t)), kp_yb/1

== system Template_v3_08_2020a/Phase #4: Return Home/Change BLACK Behavior/Hough Control ==
  Ref : Inport
  Act : Inport  Port=2
  MATLAB Function2 : MATLAB Function  TreatAsAtomicUnit=on
  MATLAB Function3 : MATLAB Function  TreatAsAtomicUnit=on
  MATLAB Function4 : MATLAB Function  TreatAsAtomicUnit=on
  Subtract2 : Sum  Inputs=+-
  Err : Outport  VectorParamsAs1DForOutWhenUnconnected=off
  wires:
  MATLAB Function4/1(e_out) -> Err/1
  MATLAB Function2/1(Oy) -> MATLAB Function4/1(Oy)
  Subtract2/1 -> MATLAB Function4/2(e_in)
  MATLAB Function2/2(Ox) -> Subtract2/1
  Act/1 -> MATLAB Function3/1(z)
  Ref/1 -> MATLAB Function2/1(z)
  MATLAB Function3/1(Ox) -> Subtract2/2

== system Template_v3_08_2020a/Phase #4: Return Home/Change BLUE Behavior/Custom Discrete PD (Attitude) ==
  ez : Inport
  Sum3 : Sum
  kd_tb : Gain  Gain=Kd_tblue
  kp_tb : Gain  Gain=Kp_tblue
  "x_dot -> x1" : Subsystem
  Tz : Outport  VectorParamsAs1DForOutWhenUnconnected=off
  wires:
  kd_tb/1 -> Sum3/1
  Sum3/1 -> Tz/1
  kp_tb/1 -> Sum3/2
  "x_dot -> x1"/1(dy(t)/dt) -> kd_tb/1
  ez/1 -> "x_dot -> x1"/1(y(t)), kp_tb/1

== system Template_v3_08_2020a/Phase #4: Return Home/Change BLUE Behavior/Custom Discrete PD (X-Position) ==
  ex : Inport
  Sum3 : Sum
  kd_xb : Gain  Gain=Kd_xblue
  kp_xb : Gain  Gain=Kp_xblue
  "x_dot -> x1" : Subsystem
  Fx : Outport  VectorParamsAs1DForOutWhenUnconnected=off
  wires:
  kd_xb/1 -> Sum3/1
  ex/1 -> "x_dot -> x1"/1(y(t)), kp_xb/1
  kp_xb/1 -> Sum3/2
  "x_dot -> x1"/1(dy(t)/dt) -> kd_xb/1
  Sum3/1 -> Fx/1

== system Template_v3_08_2020a/Phase #4: Return Home/Change BLUE Behavior/Custom Discrete PD (Y-Position) ==
  ey : Inport
  Sum3 : Sum
  kd_yb : Gain  Gain=Kd_yblue
  kp_yb : Gain  Gain=Kp_yblue
  "x_dot -> x1" : Subsystem
  Fy : Outport  VectorParamsAs1DForOutWhenUnconnected=off
  wires:
  kd_yb/1 -> Sum3/1
  Sum3/1 -> Fy/1
  kp_yb/1 -> Sum3/2
  "x_dot -> x1"/1(dy(t)/dt) -> kd_yb/1
  ey/1 -> "x_dot -> x1"/1(y(t)), kp_yb/1

== system Template_v3_08_2020a/Phase #4: Return Home/Change BLUE Behavior/Hough Control ==
  Ref : Inport
  Act : Inport  Port=2
  MATLAB Function2 : MATLAB Function  TreatAsAtomicUnit=on
  MATLAB Function3 : MATLAB Function  TreatAsAtomicUnit=on
  MATLAB Function4 : MATLAB Function  TreatAsAtomicUnit=on
  Subtract2 : Sum  Inputs=+-
  Err : Outport  VectorParamsAs1DForOutWhenUnconnected=off
  wires:
  MATLAB Function4/1(e_out) -> Err/1
  MATLAB Function2/1(Oy) -> MATLAB Function4/1(Oy)
  Subtract2/1 -> MATLAB Function4/2(e_in)
  MATLAB Function2/2(Ox) -> Subtract2/1
  Act/1 -> MATLAB Function3/1(z)
  Ref/1 -> MATLAB Function2/1(z)
  MATLAB Function3/1(Ox) -> Subtract2/2

== system Template_v3_08_2020a/Phase #4: Return Home/Change RED Behavior/Custom Discrete PD (Attitude) ==
  ez : Inport
  Sum3 : Sum
  kd_tr : Gain  Gain=Kd_tr
  kp_tr : Gain  Gain=Kp_tr
  "x_dot -> x2" : Subsystem
  Tz : Outport  VectorParamsAs1DForOutWhenUnconnected=off
  wires:
  kd_tr/1 -> Sum3/1
  Sum3/1 -> Tz/1
  kp_tr/1 -> Sum3/2
  "x_dot -> x2"/1(dy(t)/dt) -> kd_tr/1
  ez/1 -> "x_dot -> x2"/1(y(t)), kp_tr/1

== system Template_v3_08_2020a/Phase #4: Return Home/Change RED Behavior/Custom Discrete PD (X-Position) ==
  ex : Inport
  Sum3 : Sum
  kd_xr : Gain  Gain=Kd_xr
  kp_xr : Gain  Gain=Kp_xr
  "x_dot -> x2" : Subsystem
  Fx : Outport  VectorParamsAs1DForOutWhenUnconnected=off
  wires:
  kd_xr/1 -> Sum3/1
  ex/1 -> "x_dot -> x2"/1(y(t)), kp_xr/1
  kp_xr/1 -> Sum3/2
  "x_dot -> x2"/1(dy(t)/dt) -> kd_xr/1
  Sum3/1 -> Fx/1

== system Template_v3_08_2020a/Phase #4: Return Home/Change RED Behavior/Custom Discrete PD (Y-Position) ==
  ey : Inport
  Sum3 : Sum
  kd_yr : Gain  Gain=Kd_yr
  kp_yr : Gain  Gain=Kp_yr
  "x_dot -> x2" : Subsystem
  Fy : Outport  VectorParamsAs1DForOutWhenUnconnected=off
  wires:
  kd_yr/1 -> Sum3/1
  Sum3/1 -> Fy/1
  kp_yr/1 -> Sum3/2
  "x_dot -> x2"/1(dy(t)/dt) -> kd_yr/1
  ey/1 -> "x_dot -> x2"/1(y(t)), kp_yr/1

== system Template_v3_08_2020a/Phase #4: Return Home/Change RED Behavior/Hough Control ==
  Ref : Inport
  Act : Inport  Port=2
  MATLAB Function2 : MATLAB Function  TreatAsAtomicUnit=on
  MATLAB Function3 : MATLAB Function  TreatAsAtomicUnit=on
  MATLAB Function4 : MATLAB Function  TreatAsAtomicUnit=on
  Subtract2 : Sum  Inputs=+-
  Err : Outport  VectorParamsAs1DForOutWhenUnconnected=off
  wires:
  MATLAB Function4/1(e_out) -> Err/1
  MATLAB Function2/1(Oy) -> MATLAB Function4/1(Oy)
  Subtract2/1 -> MATLAB Function4/2(e_in)
  MATLAB Function2/2(Ox) -> Subtract2/1
  Act/1 -> MATLAB Function3/1(z)
  Ref/1 -> MATLAB Function2/1(z)
  MATLAB Function3/1(Ox) -> Subtract2/2

== system Template_v3_08_2020a/Phase #4: Return Home/Change RED Behavior/RED ==
  note: ARM Control Law - RED
  note: When the ARM is not in use, send zeros.
  Action Port : ActionPort  ActionPortLabel=else
  ARM_Desired_Rz_Elbow : DataStoreWrite  Commented=on  DataStoreName=ARM_Desired_Rz_Elbow
  ARM_Desired_Rz_Shoulder : DataStoreWrite  Commented=on  DataStoreName=ARM_Desired_Rz_Shoulder
  ARM_Desired_Rz_Wrist : DataStoreWrite  Commented=on  DataStoreName=ARM_Desired_Rz_Wrist
  Constant1 : Constant  Commented=on  Value=pi/2
  Constant7 : Constant  Commented=on  Value=0
  wires:
  Constant7/1 -> ARM_Desired_Rz_Wrist/1
  Constant1/1 -> ARM_Desired_Rz_Shoulder/1, ARM_Desired_Rz_Elbow/1

== system Template_v3_08_2020a/Phase #4: Return Home/Change RED Behavior/RED+ARM ==
  note: ARM Control Law - RED
  note: This section is reserved for any control law for the robotic manipulator.
  Action Port : ActionPort  ActionPortLabel=if(u1 == 4 | u1 == 5 | u1 == 10 | u1 == 11)
  Constant : Constant  Value=Phase3_End
  Data Store Read : DataStoreRead  DataStoreName=RED_Rz_Shoulder
  Data Store Read1 : DataStoreRead  DataStoreName=RED_Rz_Elbow
  Data Store Read2 : DataStoreRead  DataStoreName=RED_Rz_Wrist
  Data Store Write : DataStoreWrite  DataStoreName=RED_Shoulder_Command
  Data Store Write1 : DataStoreWrite  DataStoreName=RED_Elbow_Command
  Data Store Write2 : DataStoreWrite  DataStoreName=RED_Wrist_Command
  Data Store Write3 : DataStoreWrite  DataStoreName=RED_ARM_Control_Mode
  MATLAB Function1 : MATLAB Function  TreatAsAtomicUnit=on
  Subtract4 : Sum  Inputs=+-
  Time : DataStoreRead  DataStoreName=Univ_Time
  wires:
  Data Store Read/1 -> Data Store Write/1
  Data Store Read2/1 -> Data Store Write2/1
  Data Store Read1/1 -> Data Store Write1/1
  MATLAB Function1/1(Control_Mode) -> Data Store Write3/1
  Time/1 -> Subtract4/1
  Constant/1 -> Subtract4/2
  Subtract4/1 -> MATLAB Function1/1(Sim_Time)

== system Template_v3_08_2020a/Phase #5: Hold Home/Change BLACK Behavior/Custom Discrete PD (Attitude) ==
  ez : Inport
  Sum3 : Sum
  kd_tb : Gain  Gain=Kd_tb
  kp_tb : Gain  Gain=Kp_tb
  "x_dot -> x1" : Subsystem
  Tz : Outport  VectorParamsAs1DForOutWhenUnconnected=off
  wires:
  kd_tb/1 -> Sum3/1
  Sum3/1 -> Tz/1
  kp_tb/1 -> Sum3/2
  "x_dot -> x1"/1(dy(t)/dt) -> kd_tb/1
  ez/1 -> "x_dot -> x1"/1(y(t)), kp_tb/1

== system Template_v3_08_2020a/Phase #5: Hold Home/Change BLACK Behavior/Custom Discrete PD (X-Position) ==
  ex : Inport
  Sum3 : Sum
  kd_xb : Gain  Gain=Kd_xb
  kp_xb : Gain  Gain=Kp_xb
  "x_dot -> x1" : Subsystem
  Fx : Outport  VectorParamsAs1DForOutWhenUnconnected=off
  wires:
  kd_xb/1 -> Sum3/1
  ex/1 -> "x_dot -> x1"/1(y(t)), kp_xb/1
  kp_xb/1 -> Sum3/2
  "x_dot -> x1"/1(dy(t)/dt) -> kd_xb/1
  Sum3/1 -> Fx/1

== system Template_v3_08_2020a/Phase #5: Hold Home/Change BLACK Behavior/Custom Discrete PD (Y-Position) ==
  ey : Inport
  Sum3 : Sum
  kd_yb : Gain  Gain=Kd_yb
  kp_yb : Gain  Gain=Kp_yb
  "x_dot -> x1" : Subsystem
  Fy : Outport  VectorParamsAs1DForOutWhenUnconnected=off
  wires:
  kd_yb/1 -> Sum3/1
  Sum3/1 -> Fy/1
  kp_yb/1 -> Sum3/2
  "x_dot -> x1"/1(dy(t)/dt) -> kd_yb/1
  ey/1 -> "x_dot -> x1"/1(y(t)), kp_yb/1

== system Template_v3_08_2020a/Phase #5: Hold Home/Change BLACK Behavior/Hough Control ==
  Ref : Inport
  Act : Inport  Port=2
  MATLAB Function2 : MATLAB Function  TreatAsAtomicUnit=on
  MATLAB Function3 : MATLAB Function  TreatAsAtomicUnit=on
  MATLAB Function4 : MATLAB Function  TreatAsAtomicUnit=on
  Subtract2 : Sum  Inputs=+-
  Err : Outport  VectorParamsAs1DForOutWhenUnconnected=off
  wires:
  MATLAB Function4/1(e_out) -> Err/1
  MATLAB Function2/1(Oy) -> MATLAB Function4/1(Oy)
  Subtract2/1 -> MATLAB Function4/2(e_in)
  MATLAB Function2/2(Ox) -> Subtract2/1
  Act/1 -> MATLAB Function3/1(z)
  Ref/1 -> MATLAB Function2/1(z)
  MATLAB Function3/1(Ox) -> Subtract2/2

== system Template_v3_08_2020a/Phase #5: Hold Home/Change BLUE Behavior/Custom Discrete PD (Attitude) ==
  ez : Inport
  Sum3 : Sum
  kd_tb : Gain  Gain=Kd_tblue
  kp_tb : Gain  Gain=Kp_tblue
  "x_dot -> x1" : Subsystem
  Tz : Outport  VectorParamsAs1DForOutWhenUnconnected=off
  wires:
  kd_tb/1 -> Sum3/1
  Sum3/1 -> Tz/1
  kp_tb/1 -> Sum3/2
  "x_dot -> x1"/1(dy(t)/dt) -> kd_tb/1
  ez/1 -> "x_dot -> x1"/1(y(t)), kp_tb/1

== system Template_v3_08_2020a/Phase #5: Hold Home/Change BLUE Behavior/Custom Discrete PD (X-Position) ==
  ex : Inport
  Sum3 : Sum
  kd_xb : Gain  Gain=Kd_xblue
  kp_xb : Gain  Gain=Kp_xblue
  "x_dot -> x1" : Subsystem
  Fx : Outport  VectorParamsAs1DForOutWhenUnconnected=off
  wires:
  kd_xb/1 -> Sum3/1
  ex/1 -> "x_dot -> x1"/1(y(t)), kp_xb/1
  kp_xb/1 -> Sum3/2
  "x_dot -> x1"/1(dy(t)/dt) -> kd_xb/1
  Sum3/1 -> Fx/1

== system Template_v3_08_2020a/Phase #5: Hold Home/Change BLUE Behavior/Custom Discrete PD (Y-Position) ==
  ey : Inport
  Sum3 : Sum
  kd_yb : Gain  Gain=Kd_yblue
  kp_yb : Gain  Gain=Kp_yblue
  "x_dot -> x1" : Subsystem
  Fy : Outport  VectorParamsAs1DForOutWhenUnconnected=off
  wires:
  kd_yb/1 -> Sum3/1
  Sum3/1 -> Fy/1
  kp_yb/1 -> Sum3/2
  "x_dot -> x1"/1(dy(t)/dt) -> kd_yb/1
  ey/1 -> "x_dot -> x1"/1(y(t)), kp_yb/1

== system Template_v3_08_2020a/Phase #5: Hold Home/Change BLUE Behavior/Hough Control ==
  Ref : Inport
  Act : Inport  Port=2
  MATLAB Function2 : MATLAB Function  TreatAsAtomicUnit=on
  MATLAB Function3 : MATLAB Function  TreatAsAtomicUnit=on
  MATLAB Function4 : MATLAB Function  TreatAsAtomicUnit=on
  Subtract2 : Sum  Inputs=+-
  Err : Outport  VectorParamsAs1DForOutWhenUnconnected=off
  wires:
  MATLAB Function4/1(e_out) -> Err/1
  MATLAB Function2/1(Oy) -> MATLAB Function4/1(Oy)
  Subtract2/1 -> MATLAB Function4/2(e_in)
  MATLAB Function2/2(Ox) -> Subtract2/1
  Act/1 -> MATLAB Function3/1(z)
  Ref/1 -> MATLAB Function2/1(z)
  MATLAB Function3/1(Ox) -> Subtract2/2

== system Template_v3_08_2020a/Phase #5: Hold Home/Change RED Behavior/Custom Discrete PD (Attitude) ==
  ez : Inport
  Sum3 : Sum
  kd_tr : Gain  Gain=Kd_tr
  kp_tr : Gain  Gain=Kp_tr
  "x_dot -> x2" : Subsystem
  Tz : Outport  VectorParamsAs1DForOutWhenUnconnected=off
  wires:
  kd_tr/1 -> Sum3/1
  Sum3/1 -> Tz/1
  kp_tr/1 -> Sum3/2
  "x_dot -> x2"/1(dy(t)/dt) -> kd_tr/1
  ez/1 -> "x_dot -> x2"/1(y(t)), kp_tr/1

== system Template_v3_08_2020a/Phase #5: Hold Home/Change RED Behavior/Custom Discrete PD (X-Position) ==
  ex : Inport
  Sum3 : Sum
  kd_xr : Gain  Gain=Kd_xr
  kp_xr : Gain  Gain=Kp_xr
  "x_dot -> x2" : Subsystem
  Fx : Outport  VectorParamsAs1DForOutWhenUnconnected=off
  wires:
  kd_xr/1 -> Sum3/1
  ex/1 -> "x_dot -> x2"/1(y(t)), kp_xr/1
  kp_xr/1 -> Sum3/2
  "x_dot -> x2"/1(dy(t)/dt) -> kd_xr/1
  Sum3/1 -> Fx/1

== system Template_v3_08_2020a/Phase #5: Hold Home/Change RED Behavior/Custom Discrete PD (Y-Position) ==
  ey : Inport
  Sum3 : Sum
  kd_yr : Gain  Gain=Kd_yr
  kp_yr : Gain  Gain=Kp_yr
  "x_dot -> x2" : Subsystem
  Fy : Outport  VectorParamsAs1DForOutWhenUnconnected=off
  wires:
  kd_yr/1 -> Sum3/1
  Sum3/1 -> Fy/1
  kp_yr/1 -> Sum3/2
  "x_dot -> x2"/1(dy(t)/dt) -> kd_yr/1
  ey/1 -> "x_dot -> x2"/1(y(t)), kp_yr/1

== system Template_v3_08_2020a/Phase #5: Hold Home/Change RED Behavior/Hough Control ==
  Ref : Inport
  Act : Inport  Port=2
  MATLAB Function2 : MATLAB Function  TreatAsAtomicUnit=on
  MATLAB Function3 : MATLAB Function  TreatAsAtomicUnit=on
  MATLAB Function4 : MATLAB Function  TreatAsAtomicUnit=on
  Subtract2 : Sum  Inputs=+-
  Err : Outport  VectorParamsAs1DForOutWhenUnconnected=off
  wires:
  MATLAB Function4/1(e_out) -> Err/1
  MATLAB Function2/1(Oy) -> MATLAB Function4/1(Oy)
  Subtract2/1 -> MATLAB Function4/2(e_in)
  MATLAB Function2/2(Ox) -> Subtract2/1
  Act/1 -> MATLAB Function3/1(z)
  Ref/1 -> MATLAB Function2/1(z)
  MATLAB Function3/1(Ox) -> Subtract2/2

== system Template_v3_08_2020a/Phase #5: Hold Home/Change RED Behavior/RED ==
  note: ARM Control Law - RED
  note: When the ARM is not in use, send zeros.
  Action Port : ActionPort  ActionPortLabel=else
  ARM_Desired_Rz_Elbow : DataStoreWrite  Commented=on  DataStoreName=ARM_Desired_Rz_Elbow
  ARM_Desired_Rz_Shoulder : DataStoreWrite  Commented=on  DataStoreName=ARM_Desired_Rz_Shoulder
  ARM_Desired_Rz_Wrist : DataStoreWrite  Commented=on  DataStoreName=ARM_Desired_Rz_Wrist
  Constant1 : Constant  Commented=on  Value=pi/2
  Constant7 : Constant  Commented=on  Value=0
  wires:
  Constant7/1 -> ARM_Desired_Rz_Wrist/1
  Constant1/1 -> ARM_Desired_Rz_Shoulder/1, ARM_Desired_Rz_Elbow/1

== system Template_v3_08_2020a/Phase #5: Hold Home/Change RED Behavior/RED+ARM ==
  note: ARM Control Law - RED
  note: This section is reserved for any control law for the robotic manipulator.
  Action Port : ActionPort  ActionPortLabel=if(u1 == 4 | u1 == 5 | u1 == 10 | u1 == 11)
  Constant : Constant  Value=0
  Data Store Read : DataStoreRead  DataStoreName=RED_Rz_Shoulder
  Data Store Read1 : DataStoreRead  DataStoreName=RED_Rz_Elbow
  Data Store Read2 : DataStoreRead  DataStoreName=RED_Rz_Wrist
  Data Store Write : DataStoreWrite  DataStoreName=RED_Shoulder_Command
  Data Store Write1 : DataStoreWrite  DataStoreName=RED_Elbow_Command
  Data Store Write2 : DataStoreWrite  DataStoreName=RED_Wrist_Command
  Data Store Write3 : DataStoreWrite  DataStoreName=RED_ARM_Control_Mode
  wires:
  Data Store Read1/1 -> Data Store Write1/1
  Constant/1 -> Data Store Write3/1
  Data Store Read2/1 -> Data Store Write2/1
  Data Store Read/1 -> Data Store Write/1

== system Template_v3_08_2020a/Simulate Plant Dynamics/BLACK Dynamics/BLACK Dynamics Model ==
  control_inputs : Inport
  Acceleration to Velocity : DiscreteIntegrator  IntegratorMethod=Integration: Backward Euler  SampleTime=-1  ICPrevOutput=DiscIntNeverNeededParam  ICPrevScaledInput=DiscIntNeverNeededParam
  MATLAB Function : MATLAB Function  TreatAsAtomicUnit=on
  Random Number : RandomNumber  Variance=noise_variance_BLACK
  Sum : Sum  Inputs=|++
  Velocity to Position : DiscreteIntegrator  IntegratorMethod=Integration: Backward Euler  InitialCondition=drop_states_BLACK  SampleTime=-1  ICPrevOutput=DiscIntNeverNeededParam  ICPrevScaledInput=DiscIntNeverNeededParam
  states : Outport  VectorParamsAs1DForOutWhenUnconnected=off
  wires:
  control_inputs/1 -> MATLAB Function/1(control_inputs)
  MATLAB Function/1(x_ddot) -> Acceleration to Velocity/1
  Acceleration to Velocity/1 -> Velocity to Position/1
  Velocity to Position/1 -> Sum/1
  Sum/1 -> states/1
  Random Number/1 -> Sum/2

== system Template_v3_08_2020a/Simulate Plant Dynamics/BLACK Dynamics/Sample and Hold Data to Match PhaseSpace (BLACK) ==
  states : Inport
  Constant1 : Constant  Value=serverRate
  Data Store Read2 : DataStoreRead  DataStoreName=Univ_Time
  MATLAB Function : MATLAB Function  TreatAsAtomicUnit=on
  Sample and Hold1 : dspsigops/Sample and Hold  trig=Rising edge  initCond=drop_states_BLACK  latchinput=off
  states_hold : Outport  VectorParamsAs1DForOutWhenUnconnected=off
  wires:
  states/1 -> Sample and Hold1/1
  Data Store Read2/1 -> MATLAB Function/1(TIME)
  Constant1/1 -> MATLAB Function/2(SERVER)
  MATLAB Function/1(y) -> Sample and Hold1/Trigger
  Sample and Hold1/1 -> states_hold/1

== system Template_v3_08_2020a/Simulate Plant Dynamics/BLACK Dynamics/x_dot -> x1 ==
  note: dy/dt ~= (y2-y1)/deltaT
  y(t) : Inport
  Delay1 : Delay  DelayLength=1  InitialConditionSource=Input port
      settings: InputPortMap=u0,p4
  Hold this value : Subsystem  TreatAsAtomicUnit=on
  Sum6 : Sum  Inputs=-+|
  divide by delta T : Gain  Gain=1/baseRate
  "if we went through a \"step\"" : If  IfExpression=u1 ~= 0  ShowElse=off
  dy(t)/dt : Outport  VectorParamsAs1DForOutWhenUnconnected=off
  wires:
  divide by delta T/1 -> dy(t)/dt/1
  Delay1/1 -> Sum6/1
  "if we went through a \"step\""/1 -> Hold this value/Action
  Hold this value/1(Out1) -> divide by delta T/1
  Sum6/1 -> "if we went through a \"step\""/1, Hold this value/1(In1)
  y(t)/1 -> Sum6/2, Delay1/2, Delay1/1

== system Template_v3_08_2020a/Simulate Plant Dynamics/BLACK Dynamics/x_dot -> x2 ==
  note: dy/dt ~= (y2-y1)/deltaT
  y(t) : Inport
  Delay1 : Delay  DelayLength=1  InitialConditionSource=Input port
      settings: InputPortMap=u0,p4
  Hold this value : Subsystem  TreatAsAtomicUnit=on
  Sum6 : Sum  Inputs=-+|
  divide by delta T : Gain  Gain=1/baseRate
  "if we went through a \"step\"" : If  IfExpression=u1 ~= 0  ShowElse=off
  dy(t)/dt : Outport  VectorParamsAs1DForOutWhenUnconnected=off
  wires:
  divide by delta T/1 -> dy(t)/dt/1
  Delay1/1 -> Sum6/1
  "if we went through a \"step\""/1 -> Hold this value/Action
  Hold this value/1(Out1) -> divide by delta T/1
  Sum6/1 -> "if we went through a \"step\""/1, Hold this value/1(In1)
  y(t)/1 -> Sum6/2, Delay1/2, Delay1/1
